simulink library "z5234550RundongGuanLib_DT1_2020"  (R2020a)
settings: Solver=VariableStepAuto  StartTime=0.0  StopTime=10.0  RelTol=1e-3
values from neighbouring files (symbols this model uses):
  Tcs = 1e-4    (= 0.0001)    [z5234550RundongGuanInit_DT1_2020.m]    (also in z5234550RundongGuanSOGIBODE_DT1_2020.m; z5234550RundongGuanTestKiKp_DT1_2020.m; z5234550RundongGuanTestKi_DT1_2020.m; z5234550RundongGuanTestKp_DT1_2020.m)
undefined symbols (not defined in the file or in its folder): DiscIntNeverNeededParam
libraries: $bdroot x6, simulink x5
settings Model: Creator=Kevin  LastModifiedBy=Kevin

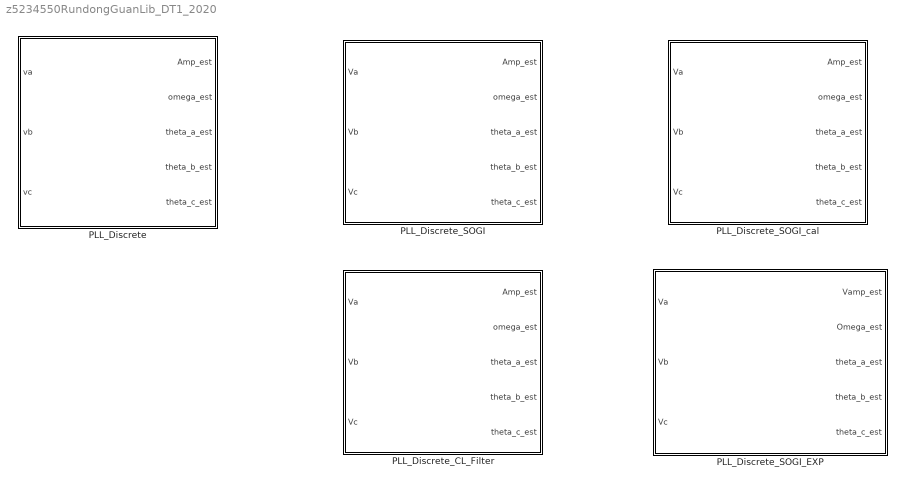
== system z5234550RundongGuanLib_DT1_2020 ==
  PLL_Discrete : Subsystem
  PLL_Discrete_CL_Filter : Subsystem
  PLL_Discrete_SOGI : Subsystem
  PLL_Discrete_SOGI_EXP : Subsystem
  PLL_Discrete_SOGI_cal : Subsystem

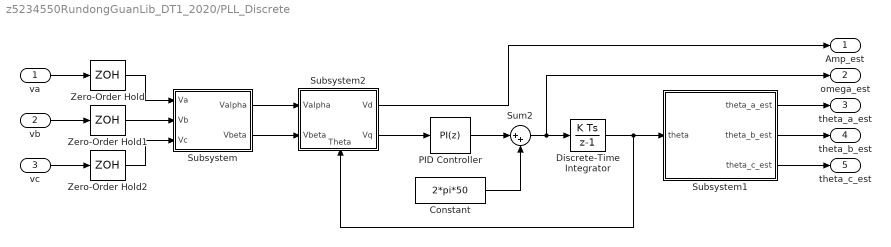
== system z5234550RundongGuanLib_DT1_2020/PLL_Discrete ==
  va : Inport
  vb : Inport  Port=2
  vc : Inport  Port=3
  Constant : Constant  Value=2*pi*50  SampleTime=Tcs
  Discrete-Time Integrator : DiscreteIntegrator  SampleTime=Tcs  ICPrevOutput=DiscIntNeverNeededParam  ICPrevScaledInput=DiscIntNeverNeededParam
  PID Controller : simulink/Continuous/PID Controller  Controller=PI  Form=Parallel  TimeDomain=Discrete-time  UseExternalTs=off  SampleTime=Tcs  IntegratorMethod=Forward Euler  FilterMethod=Forward Euler  ControllerParametersSource=internal  P=4.1744  I=2322.32  D=0  UseFilter=on  N=100  TunerSelectOption=Transfer Function Based (PID Tuner App)  InitialConditionSource=internal  InitialConditionForIntegrator=0  InitialConditionForFilter=0  DifferentiatorICPrevScaledInput=0  ExternalReset=none  TrackingMode=off  Kt=1  LimitOutput=off  UpperSaturationLimit=inf  LowerSaturationLimit=-inf  LinearizeAsGain=on  AntiWindupMode=none  Kb=1  POutMin=[]  POutMax=[]  IOutMin=[]  IOutMax=[]  DOutMin=[]  DOutMax=[]  NOutMin=[]  NOutMax=[]  SumOutMin=[]  SumOutMax=[]  SaturationOutMin=[]  SaturationOutMax=[]  PParamMin=[]  PParamMax=[]  IParamMin=[]  IParamMax=[]  DParamMin=[]  DParamMax=[]  NParamMin=[]  NParamMax=[]  KbParamMin=[]  KbParamMax=[]  KtParamMin=[]  KtParamMax=[]  KbOutMin=[]  KbOutMax=[]  KtOutMin=[]  KtOutMax=[]  IntegratorOutMin=[]  IntegratorOutMax=[]  FilterOutMin=[]  FilterOutMax=[]  SumI1OutMin=[]  SumI1OutMax=[]  SumI2OutMin=[]  SumI2OutMax=[]  SumI3OutMin=[]  SumI3OutMax=[]  SumI4OutMin=[]  SumI4OutMax=[]  SumDOutMin=[]  SumDOutMax=[]  DifferentiatorOutMin=[]  DifferentiatorOutMax=[]  FilterDiffOutCoefMin=[]  FilterDiffOutCoefMax=[]  ReciprocalOutMin=[]  ReciprocalOutMax=[]  SumDenOutMin=[]  SumDenOutMax=[]  SumNumOutMin=[]  SumNumOutMax=[]  DivideOutMin=[]  DivideOutMax=[]  UdiffTsProdOutMin=[]  UdiffTsProdOutMax=[]  NTsProdOutMin=[]  NTsProdOutMax=[]  UintegralTsProdOutMin=[]  UintegralTsProdOutMax=[]  UngainTsProdOutMin=[]  UngainTsProdOutMax=[]  IntegratorContinuousStateAttributes=''  IntegratorStateMustResolveToSignalObject=off  IntegratorRTWStateStorageClass=Auto  FilterContinuousStateAttributes=''  FilterStateMustResolveToSignalObject=off  FilterRTWStateStorageClass=Auto  ParallelPVariant=InternalParameters  IdealPVariant=Disabled  IVariant=InternalParameters  DVariant=Disabled  IntegratorVariant=Discrete  SatVariant=Disabled  AWVariant=Passthrough  PCopyVariant=Disabled  TRVariant=Disabled  FdbkBlocksVariant=Forward  IdealPFdbkVariant=Disabled  SatFdbkVariant=Disabled  DerivativeFilterVariant=Disabled  NVariant=Disabled  NCopyVariant=Disabled_SignalSpec  FilterICVariant=Disabled  IntegratorICVariant=InternalICs  ExternalResetVariant=Disabled  TRSumVariant=Passthrough  SumFdbkVariant=Disabled  SumVariant=Sum_PI  TsampFilterVariant=InternalTs  TsampNgainVariant=Passthrough  TsampIntegralVariant=Passthrough
  Subsystem : Subsystem
  Subsystem1 : Subsystem
  Subsystem2 : Subsystem
      settings: PortSchema="{\"entries\":[{\"content\":{\"sides\":[{\"content\":{\"connectorIds\":[\"In1\",\"In2\"]},\"type\":\"ConnectorPlacement.EquallySpacedRectSide\",\"uuid\":\"d7ee73cc-3741-4077-b32c-689f2c701f83\"},{\"content\":{\"connectorIds\":[\"Out1\",\"Out2\"],\"side\":\"RIGHT\"},\"type\":\"ConnectorPlacement.EquallySpacedRectSide\",\"uuid\":\"fa84044a-ecd8-49d8-a4b2-ae549d89fe8f\"},{\"content\":{\"connectorIds\":[],\"side\":\"TOP\"},\"type\":\"ConnectorPlacement.EquallySpacedRectSide\",\"uuid\":\"692e7773-1833-4597-a5fd-7846ecf4550e\"},{\"content\":{\"connectorIds\":[\"In3\"],\"side\":\"BOTTOM\"},\"type\":\"ConnectorPlacement.EquallySpacedRectSide\",\"uuid\":\"73d654b9-9f56-4244-9824-eb13bf44a38f\"}]},\"type\":\"ConnectorPlacement.EquallySpacedConnector\",\"uuid\":\"4e0b4972-389e-416e-b0d9-9fdc8ba0f1f7\"}],\"packageUris\":[\"http://schema.mathworks.com/mf0/Connector/19700101\"],\"version\":\"1.0\"}"
  Sum2 : Sum  Inputs=|++
  Zero-Order Hold : ZeroOrderHold  SampleTime=Tcs
  Zero-Order Hold1 : ZeroOrderHold  SampleTime=Tcs
  Zero-Order Hold2 : ZeroOrderHold  SampleTime=Tcs
  Amp_est : Outport
  omega_est : Outport  Port=2
  theta_a_est : Outport  Port=3
  theta_b_est : Outport  Port=4
  theta_c_est : Outport  Port=5
  wires:
  va/1 -> Zero-Order Hold/1
  vb/1 -> Zero-Order Hold1/1
  vc/1 -> Zero-Order Hold2/1
  Zero-Order Hold/1 -> Subsystem/1(Va)
  Zero-Order Hold2/1 -> Subsystem/3(Vc)
  Zero-Order Hold1/1 -> Subsystem/2(Vb)
  Subsystem/2(Vbeta) -> Subsystem2/2(Vbeta)
  Subsystem/1(Valpha) -> Subsystem2/1(Valpha)
  PID Controller/1 -> Sum2/1
  Subsystem2/1(Vd) -> Amp_est/1
  Constant/1 -> Sum2/2
  Subsystem1/1(theta_a_est) -> theta_a_est/1
  Subsystem1/2(theta_b_est) -> theta_b_est/1
  Subsystem1/3(theta_c_est) -> theta_c_est/1
  Subsystem2/2(Vq) -> PID Controller/1
  Sum2/1 -> Discrete-Time Integrator/1, omega_est/1
  Discrete-Time Integrator/1 -> Subsystem1/1(theta), Subsystem2/3(Theta)

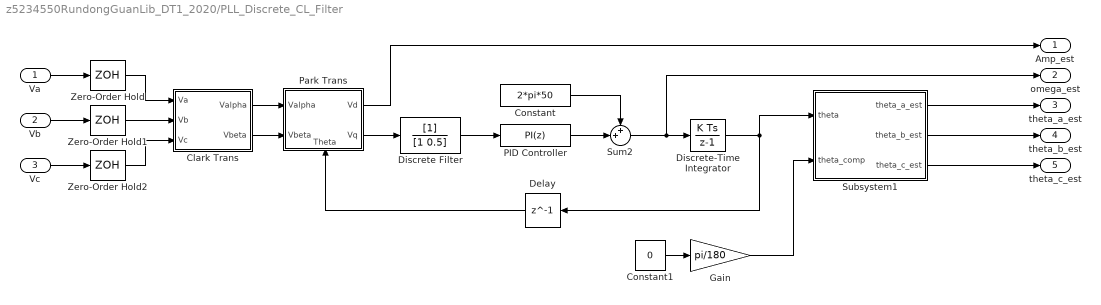
== system z5234550RundongGuanLib_DT1_2020/PLL_Discrete_CL_Filter ==
  Va : Inport
  Vb : Inport  Port=2
  Vc : Inport  Port=3
  Clark Trans : Subsystem
  Constant : Constant  Value=2*pi*50  SampleTime=Tcs
  Constant1 : Constant  Value=0
  Delay : Delay  DelayLength=1  SampleTime=Tcs
  Discrete Filter : DiscreteFilter
  Discrete-Time Integrator : DiscreteIntegrator  SampleTime=Tcs  ICPrevOutput=DiscIntNeverNeededParam  ICPrevScaledInput=DiscIntNeverNeededParam
  Gain : Gain  Gain=pi/180
  PID Controller : simulink/Continuous/PID Controller  Controller=PI  Form=Parallel  TimeDomain=Discrete-time  UseExternalTs=off  SampleTime=Tcs  IntegratorMethod=Forward Euler  FilterMethod=Forward Euler  ControllerParametersSource=internal  P=5.1744  I=0.01  D=0  UseFilter=on  N=100  TunerSelectOption=Transfer Function Based (PID Tuner App)  InitialConditionSource=internal  InitialConditionForIntegrator=0  InitialConditionForFilter=0  DifferentiatorICPrevScaledInput=0  ExternalReset=none  TrackingMode=off  Kt=1  LimitOutput=off  UpperSaturationLimit=inf  LowerSaturationLimit=-inf  LinearizeAsGain=on  AntiWindupMode=none  Kb=1  POutMin=[]  POutMax=[]  IOutMin=[]  IOutMax=[]  DOutMin=[]  DOutMax=[]  NOutMin=[]  NOutMax=[]  SumOutMin=[]  SumOutMax=[]  SaturationOutMin=[]  SaturationOutMax=[]  PParamMin=[]  PParamMax=[]  IParamMin=[]  IParamMax=[]  DParamMin=[]  DParamMax=[]  NParamMin=[]  NParamMax=[]  KbParamMin=[]  KbParamMax=[]  KtParamMin=[]  KtParamMax=[]  KbOutMin=[]  KbOutMax=[]  KtOutMin=[]  KtOutMax=[]  IntegratorOutMin=[]  IntegratorOutMax=[]  FilterOutMin=[]  FilterOutMax=[]  SumI1OutMin=[]  SumI1OutMax=[]  SumI2OutMin=[]  SumI2OutMax=[]  SumI3OutMin=[]  SumI3OutMax=[]  SumI4OutMin=[]  SumI4OutMax=[]  SumDOutMin=[]  SumDOutMax=[]  DifferentiatorOutMin=[]  DifferentiatorOutMax=[]  FilterDiffOutCoefMin=[]  FilterDiffOutCoefMax=[]  ReciprocalOutMin=[]  ReciprocalOutMax=[]  SumDenOutMin=[]  SumDenOutMax=[]  SumNumOutMin=[]  SumNumOutMax=[]  DivideOutMin=[]  DivideOutMax=[]  UdiffTsProdOutMin=[]  UdiffTsProdOutMax=[]  NTsProdOutMin=[]  NTsProdOutMax=[]  UintegralTsProdOutMin=[]  UintegralTsProdOutMax=[]  UngainTsProdOutMin=[]  UngainTsProdOutMax=[]  IntegratorContinuousStateAttributes=''  IntegratorStateMustResolveToSignalObject=off  IntegratorRTWStateStorageClass=Auto  FilterContinuousStateAttributes=''  FilterStateMustResolveToSignalObject=off  FilterRTWStateStorageClass=Auto  ParallelPVariant=InternalParameters  IdealPVariant=Disabled  IVariant=InternalParameters  DVariant=Disabled  IntegratorVariant=Discrete  SatVariant=Disabled  AWVariant=Passthrough  PCopyVariant=Disabled  TRVariant=Disabled  FdbkBlocksVariant=Forward  IdealPFdbkVariant=Disabled  SatFdbkVariant=Disabled  DerivativeFilterVariant=Disabled  NVariant=Disabled  NCopyVariant=Disabled_SignalSpec  FilterICVariant=Disabled  IntegratorICVariant=InternalICs  ExternalResetVariant=Disabled  TRSumVariant=Passthrough  SumFdbkVariant=Disabled  SumVariant=Sum_PI  TsampFilterVariant=InternalTs  TsampNgainVariant=Passthrough  TsampIntegralVariant=Passthrough
  Park Trans : Subsystem
      settings: PortSchema="{\"entries\":[{\"content\":{\"sides\":[{\"content\":{\"connectorIds\":[\"In1\",\"In2\"]},\"type\":\"ConnectorPlacement.EquallySpacedRectSide\",\"uuid\":\"d7ee73cc-3741-4077-b32c-689f2c701f83\"},{\"content\":{\"connectorIds\":[\"Out1\",\"Out2\"],\"side\":\"RIGHT\"},\"type\":\"ConnectorPlacement.EquallySpacedRectSide\",\"uuid\":\"fa84044a-ecd8-49d8-a4b2-ae549d89fe8f\"},{\"content\":{\"connectorIds\":[],\"side\":\"TOP\"},\"type\":\"ConnectorPlacement.EquallySpacedRectSide\",\"uuid\":\"692e7773-1833-4597-a5fd-7846ecf4550e\"},{\"content\":{\"connectorIds\":[\"In3\"],\"side\":\"BOTTOM\"},\"type\":\"ConnectorPlacement.EquallySpacedRectSide\",\"uuid\":\"73d654b9-9f56-4244-9824-eb13bf44a38f\"}]},\"type\":\"ConnectorPlacement.EquallySpacedConnector\",\"uuid\":\"4e0b4972-389e-416e-b0d9-9fdc8ba0f1f7\"}],\"packageUris\":[\"http://schema.mathworks.com/mf0/Connector/19700101\"],\"version\":\"1.0\"}"
  Subsystem1 : Subsystem
  Sum2 : Sum  Inputs=++|
  Zero-Order Hold : ZeroOrderHold  SampleTime=Tcs
  Zero-Order Hold1 : ZeroOrderHold  SampleTime=Tcs
  Zero-Order Hold2 : ZeroOrderHold  SampleTime=Tcs
  Amp_est : Outport
  omega_est : Outport  Port=2
  theta_a_est : Outport  Port=3
  theta_b_est : Outport  Port=4
  theta_c_est : Outport  Port=5
  wires:
  Zero-Order Hold1/1 -> Clark Trans/2(Vb)
  Vc/1 -> Zero-Order Hold2/1
  Vb/1 -> Zero-Order Hold1/1
  Zero-Order Hold2/1 -> Clark Trans/3(Vc)
  Zero-Order Hold/1 -> Clark Trans/1(Va)
  Va/1 -> Zero-Order Hold/1
  Subsystem1/1(theta_a_est) -> theta_a_est/1
  Subsystem1/2(theta_b_est) -> theta_b_est/1
  Subsystem1/3(theta_c_est) -> theta_c_est/1
  Sum2/1 -> Discrete-Time Integrator/1, omega_est/1
  Clark Trans/1(Valpha) -> Park Trans/1(Valpha)
  Clark Trans/2(Vbeta) -> Park Trans/2(Vbeta)
  Delay/1 -> Park Trans/3(Theta)
  PID Controller/1 -> Sum2/2
  Constant/1 -> Sum2/1
  Discrete-Time Integrator/1 -> Subsystem1/1(theta), Delay/1
  Park Trans/1(Vd) -> Amp_est/1
  Constant1/1 -> Gain/1
  Gain/1 -> Subsystem1/2(theta_comp)
  Park Trans/2(Vq) -> Discrete Filter/1
  Discrete Filter/1 -> PID Controller/1

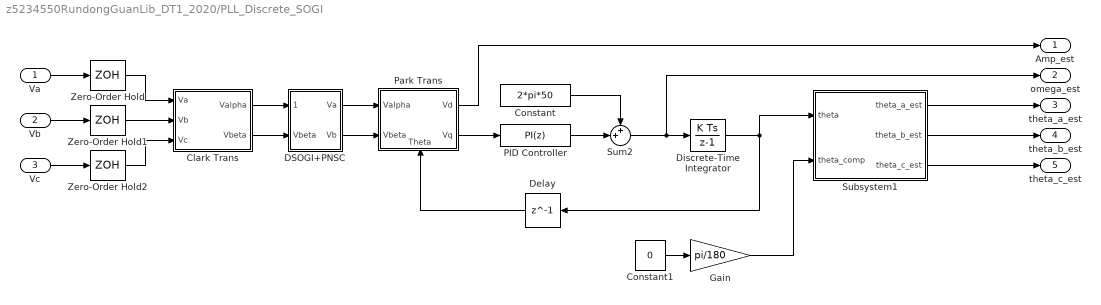
== system z5234550RundongGuanLib_DT1_2020/PLL_Discrete_SOGI ==
  Va : Inport
  Vb : Inport  Port=2
  Vc : Inport  Port=3
  Clark Trans : Subsystem
  Constant : Constant  Value=2*pi*50  SampleTime=Tcs
  Constant1 : Constant  Value=0
  DSOGI+PNSC : Subsystem
  Delay : Delay  DelayLength=1  SampleTime=Tcs
  Discrete-Time Integrator : DiscreteIntegrator  SampleTime=Tcs  ICPrevOutput=DiscIntNeverNeededParam  ICPrevScaledInput=DiscIntNeverNeededParam
  Gain : Gain  Gain=pi/180
  PID Controller : simulink/Continuous/PID Controller  Controller=PI  Form=Parallel  TimeDomain=Discrete-time  UseExternalTs=off  SampleTime=Tcs  IntegratorMethod=Forward Euler  FilterMethod=Forward Euler  ControllerParametersSource=internal  P=5.1744  I=100  D=0  UseFilter=on  N=100  TunerSelectOption=Transfer Function Based (PID Tuner App)  InitialConditionSource=internal  InitialConditionForIntegrator=0  InitialConditionForFilter=0  DifferentiatorICPrevScaledInput=0  ExternalReset=none  TrackingMode=off  Kt=1  LimitOutput=off  UpperSaturationLimit=inf  LowerSaturationLimit=-inf  LinearizeAsGain=on  AntiWindupMode=none  Kb=1  POutMin=[]  POutMax=[]  IOutMin=[]  IOutMax=[]  DOutMin=[]  DOutMax=[]  NOutMin=[]  NOutMax=[]  SumOutMin=[]  SumOutMax=[]  SaturationOutMin=[]  SaturationOutMax=[]  PParamMin=[]  PParamMax=[]  IParamMin=[]  IParamMax=[]  DParamMin=[]  DParamMax=[]  NParamMin=[]  NParamMax=[]  KbParamMin=[]  KbParamMax=[]  KtParamMin=[]  KtParamMax=[]  KbOutMin=[]  KbOutMax=[]  KtOutMin=[]  KtOutMax=[]  IntegratorOutMin=[]  IntegratorOutMax=[]  FilterOutMin=[]  FilterOutMax=[]  SumI1OutMin=[]  SumI1OutMax=[]  SumI2OutMin=[]  SumI2OutMax=[]  SumI3OutMin=[]  SumI3OutMax=[]  SumI4OutMin=[]  SumI4OutMax=[]  SumDOutMin=[]  SumDOutMax=[]  DifferentiatorOutMin=[]  DifferentiatorOutMax=[]  FilterDiffOutCoefMin=[]  FilterDiffOutCoefMax=[]  ReciprocalOutMin=[]  ReciprocalOutMax=[]  SumDenOutMin=[]  SumDenOutMax=[]  SumNumOutMin=[]  SumNumOutMax=[]  DivideOutMin=[]  DivideOutMax=[]  UdiffTsProdOutMin=[]  UdiffTsProdOutMax=[]  NTsProdOutMin=[]  NTsProdOutMax=[]  UintegralTsProdOutMin=[]  UintegralTsProdOutMax=[]  UngainTsProdOutMin=[]  UngainTsProdOutMax=[]  IntegratorContinuousStateAttributes=''  IntegratorStateMustResolveToSignalObject=off  IntegratorRTWStateStorageClass=Auto  FilterContinuousStateAttributes=''  FilterStateMustResolveToSignalObject=off  FilterRTWStateStorageClass=Auto  ParallelPVariant=InternalParameters  IdealPVariant=Disabled  IVariant=InternalParameters  DVariant=Disabled  IntegratorVariant=Discrete  SatVariant=Disabled  AWVariant=Passthrough  PCopyVariant=Disabled  TRVariant=Disabled  FdbkBlocksVariant=Forward  IdealPFdbkVariant=Disabled  SatFdbkVariant=Disabled  DerivativeFilterVariant=Disabled  NVariant=Disabled  NCopyVariant=Disabled_SignalSpec  FilterICVariant=Disabled  IntegratorICVariant=InternalICs  ExternalResetVariant=Disabled  TRSumVariant=Passthrough  SumFdbkVariant=Disabled  SumVariant=Sum_PI  TsampFilterVariant=InternalTs  TsampNgainVariant=Passthrough  TsampIntegralVariant=Passthrough
  Park Trans : Subsystem
      settings: PortSchema="{\"entries\":[{\"content\":{\"sides\":[{\"content\":{\"connectorIds\":[\"In1\",\"In2\"]},\"type\":\"ConnectorPlacement.EquallySpacedRectSide\",\"uuid\":\"d7ee73cc-3741-4077-b32c-689f2c701f83\"},{\"content\":{\"connectorIds\":[\"Out1\",\"Out2\"],\"side\":\"RIGHT\"},\"type\":\"ConnectorPlacement.EquallySpacedRectSide\",\"uuid\":\"fa84044a-ecd8-49d8-a4b2-ae549d89fe8f\"},{\"content\":{\"connectorIds\":[],\"side\":\"TOP\"},\"type\":\"ConnectorPlacement.EquallySpacedRectSide\",\"uuid\":\"692e7773-1833-4597-a5fd-7846ecf4550e\"},{\"content\":{\"connectorIds\":[\"In3\"],\"side\":\"BOTTOM\"},\"type\":\"ConnectorPlacement.EquallySpacedRectSide\",\"uuid\":\"73d654b9-9f56-4244-9824-eb13bf44a38f\"}]},\"type\":\"ConnectorPlacement.EquallySpacedConnector\",\"uuid\":\"4e0b4972-389e-416e-b0d9-9fdc8ba0f1f7\"}],\"packageUris\":[\"http://schema.mathworks.com/mf0/Connector/19700101\"],\"version\":\"1.0\"}"
  Subsystem1 : Subsystem
  Sum2 : Sum  Inputs=++|
  Zero-Order Hold : ZeroOrderHold  SampleTime=Tcs
  Zero-Order Hold1 : ZeroOrderHold  SampleTime=Tcs
  Zero-Order Hold2 : ZeroOrderHold  SampleTime=Tcs
  Amp_est : Outport
  omega_est : Outport  Port=2
  theta_a_est : Outport  Port=3
  theta_b_est : Outport  Port=4
  theta_c_est : Outport  Port=5
  wires:
  Zero-Order Hold1/1 -> Clark Trans/2(Vb)
  Vc/1 -> Zero-Order Hold2/1
  Vb/1 -> Zero-Order Hold1/1
  Zero-Order Hold2/1 -> Clark Trans/3(Vc)
  Zero-Order Hold/1 -> Clark Trans/1(Va)
  Va/1 -> Zero-Order Hold/1
  Subsystem1/1(theta_a_est) -> theta_a_est/1
  Subsystem1/2(theta_b_est) -> theta_b_est/1
  Subsystem1/3(theta_c_est) -> theta_c_est/1
  Sum2/1 -> Discrete-Time Integrator/1, omega_est/1
  Park Trans/2(Vq) -> PID Controller/1
  Clark Trans/1(Valpha) -> DSOGI+PNSC/1(Valpha)
  Clark Trans/2(Vbeta) -> DSOGI+PNSC/2(Vbeta)
  DSOGI+PNSC/1(Va) -> Park Trans/1(Valpha)
  DSOGI+PNSC/2(Vb) -> Park Trans/2(Vbeta)
  Delay/1 -> Park Trans/3(Theta)
  PID Controller/1 -> Sum2/2
  Constant/1 -> Sum2/1
  Discrete-Time Integrator/1 -> Subsystem1/1(theta), Delay/1
  Park Trans/1(Vd) -> Amp_est/1
  Constant1/1 -> Gain/1
  Gain/1 -> Subsystem1/2(theta_comp)

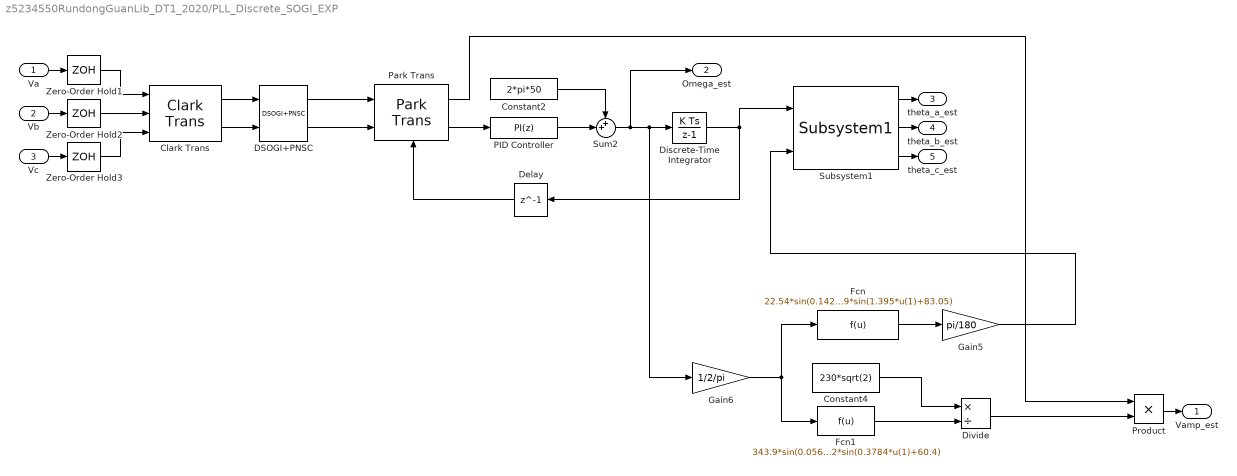
== system z5234550RundongGuanLib_DT1_2020/PLL_Discrete_SOGI_EXP ==
  Va : Inport
  Vb : Inport  Port=2
  Vc : Inport  Port=3
  Clark Trans : $bdroot/PLL_Discrete_SOGI/Clark Trans  SystemSampleTime=-1  Latency=0  AutoFrameSizeCalculation=off
  Constant2 : Constant  Value=2*pi*50  SampleTime=Tcs
  Constant4 : Constant  Value=230*sqrt(2)
  DSOGI+PNSC : $bdroot/PLL_Discrete_SOGI/DSOGI+PNSC  SystemSampleTime=-1  Latency=0  AutoFrameSizeCalculation=off
      link override Subsystem1/Gain: Gain=0.75
      link override Subsystem3/Gain: Gain=0.75
  Delay : Delay  DelayLength=1  SampleTime=Tcs
  Discrete-Time Integrator : DiscreteIntegrator  SampleTime=Tcs  ICPrevOutput=DiscIntNeverNeededParam  ICPrevScaledInput=DiscIntNeverNeededParam
  Divide : Product  Inputs=*/
  Fcn : Fcn  Expr=22.54*sin(0.1425*u(1)+68.25)+0.07009*sin(1.395*u(1)+83.05)
  Fcn1 : Fcn  Expr=343.9*sin(0.05621*u(1)+36.6)+1.732*sin(0.3784*u(1)+60.4)
  Gain5 : Gain  Gain=pi/180
  Gain6 : Gain  Gain=1/2/pi
  PID Controller : simulink/Continuous/PID Controller  Controller=PI  Form=Parallel  TimeDomain=Discrete-time  UseExternalTs=off  SampleTime=Tcs  IntegratorMethod=Forward Euler  FilterMethod=Forward Euler  ControllerParametersSource=internal  P=4  I=100  D=0  UseFilter=on  N=100  TunerSelectOption=Transfer Function Based (PID Tuner App)  InitialConditionSource=internal  InitialConditionForIntegrator=0  InitialConditionForFilter=0  DifferentiatorICPrevScaledInput=0  ExternalReset=none  TrackingMode=off  Kt=1  LimitOutput=off  UpperSaturationLimit=inf  LowerSaturationLimit=-inf  LinearizeAsGain=on  AntiWindupMode=none  Kb=1  POutMin=[]  POutMax=[]  IOutMin=[]  IOutMax=[]  DOutMin=[]  DOutMax=[]  NOutMin=[]  NOutMax=[]  SumOutMin=[]  SumOutMax=[]  SaturationOutMin=[]  SaturationOutMax=[]  PParamMin=[]  PParamMax=[]  IParamMin=[]  IParamMax=[]  DParamMin=[]  DParamMax=[]  NParamMin=[]  NParamMax=[]  KbParamMin=[]  KbParamMax=[]  KtParamMin=[]  KtParamMax=[]  KbOutMin=[]  KbOutMax=[]  KtOutMin=[]  KtOutMax=[]  IntegratorOutMin=[]  IntegratorOutMax=[]  FilterOutMin=[]  FilterOutMax=[]  SumI1OutMin=[]  SumI1OutMax=[]  SumI2OutMin=[]  SumI2OutMax=[]  SumI3OutMin=[]  SumI3OutMax=[]  SumI4OutMin=[]  SumI4OutMax=[]  SumDOutMin=[]  SumDOutMax=[]  DifferentiatorOutMin=[]  DifferentiatorOutMax=[]  FilterDiffOutCoefMin=[]  FilterDiffOutCoefMax=[]  ReciprocalOutMin=[]  ReciprocalOutMax=[]  SumDenOutMin=[]  SumDenOutMax=[]  SumNumOutMin=[]  SumNumOutMax=[]  DivideOutMin=[]  DivideOutMax=[]  UdiffTsProdOutMin=[]  UdiffTsProdOutMax=[]  NTsProdOutMin=[]  NTsProdOutMax=[]  UintegralTsProdOutMin=[]  UintegralTsProdOutMax=[]  UngainTsProdOutMin=[]  UngainTsProdOutMax=[]  IntegratorContinuousStateAttributes=''  IntegratorStateMustResolveToSignalObject=off  IntegratorRTWStateStorageClass=Auto  FilterContinuousStateAttributes=''  FilterStateMustResolveToSignalObject=off  FilterRTWStateStorageClass=Auto  ParallelPVariant=InternalParameters  IdealPVariant=Disabled  IVariant=InternalParameters  DVariant=Disabled  IntegratorVariant=Discrete  SatVariant=Disabled  AWVariant=Passthrough  PCopyVariant=Disabled  TRVariant=Disabled  FdbkBlocksVariant=Forward  IdealPFdbkVariant=Disabled  SatFdbkVariant=Disabled  DerivativeFilterVariant=Disabled  NVariant=Disabled  NCopyVariant=Disabled_SignalSpec  FilterICVariant=Disabled  IntegratorICVariant=InternalICs  ExternalResetVariant=Disabled  TRSumVariant=Passthrough  SumFdbkVariant=Disabled  SumVariant=Sum_PI  TsampFilterVariant=InternalTs  TsampNgainVariant=Passthrough  TsampIntegralVariant=Passthrough
  Park Trans : $bdroot/PLL_Discrete_SOGI/Park Trans  SystemSampleTime=-1  Latency=0  AutoFrameSizeCalculation=off
      settings: PortSchema="{\"entries\":[{\"content\":{\"sides\":[{\"content\":{\"connectorIds\":[\"In1\",\"In2\"]},\"type\":\"ConnectorPlacement.EquallySpacedRectSide\",\"uuid\":\"d7ee73cc-3741-4077-b32c-689f2c701f83\"},{\"content\":{\"connectorIds\":[\"Out1\",\"Out2\"],\"side\":\"RIGHT\"},\"type\":\"ConnectorPlacement.EquallySpacedRectSide\",\"uuid\":\"fa84044a-ecd8-49d8-a4b2-ae549d89fe8f\"},{\"content\":{\"connectorIds\":[],\"side\":\"TOP\"},\"type\":\"ConnectorPlacement.EquallySpacedRectSide\",\"uuid\":\"692e7773-1833-4597-a5fd-7846ecf4550e\"},{\"content\":{\"connectorIds\":[\"In3\"],\"side\":\"BOTTOM\"},\"type\":\"ConnectorPlacement.EquallySpacedRectSide\",\"uuid\":\"73d654b9-9f56-4244-9824-eb13bf44a38f\"}]},\"type\":\"ConnectorPlacement.EquallySpacedConnector\",\"uuid\":\"4e0b4972-389e-416e-b0d9-9fdc8ba0f1f7\"}],\"packageUris\":[\"http://schema.mathworks.com/mf0/Connector/19700101\"],\"version\":\"1.0\"}"
  Product : Product
  Subsystem1 : $bdroot/PLL_Discrete_SOGI/Subsystem1  SystemSampleTime=-1  Latency=0  AutoFrameSizeCalculation=off
  Sum2 : Sum  Inputs=++|
  Zero-Order Hold1 : ZeroOrderHold  SampleTime=Tcs
  Zero-Order Hold2 : ZeroOrderHold  SampleTime=Tcs
  Zero-Order Hold3 : ZeroOrderHold  SampleTime=Tcs
  Vamp_est : Outport
  Omega_est : Outport  Port=2
  theta_a_est : Outport  Port=3
  theta_b_est : Outport  Port=4
  theta_c_est : Outport  Port=5
  wires:
  Fcn/1 -> Gain5/1
  Gain5/1 -> Subsystem1/2
  Gain6/1 -> Fcn1/1, Fcn/1
  Constant2/1 -> Sum2/1
  Clark Trans/1 -> DSOGI+PNSC/1
  Constant4/1 -> Divide/1
  Fcn1/1 -> Divide/2
  Discrete-Time Integrator/1 -> Subsystem1/1, Delay/1
  Zero-Order Hold1/1 -> Clark Trans/1
  DSOGI+PNSC/1 -> Park Trans/1
  DSOGI+PNSC/2 -> Park Trans/2
  Va/1 -> Zero-Order Hold1/1
  Park Trans/1 -> Product/1
  Zero-Order Hold3/1 -> Clark Trans/3
  PID Controller/1 -> Sum2/2
  Subsystem1/2 -> theta_b_est/1
  Vb/1 -> Zero-Order Hold2/1
  Subsystem1/1 -> theta_a_est/1
  Zero-Order Hold2/1 -> Clark Trans/2
  Sum2/1 -> Omega_est/1, Gain6/1, Discrete-Time Integrator/1
  Clark Trans/2 -> DSOGI+PNSC/2
  Product/1 -> Vamp_est/1
  Delay/1 -> Park Trans/3
  Park Trans/2 -> PID Controller/1
  Divide/1 -> Product/2
  Vc/1 -> Zero-Order Hold3/1
  Subsystem1/3 -> theta_c_est/1

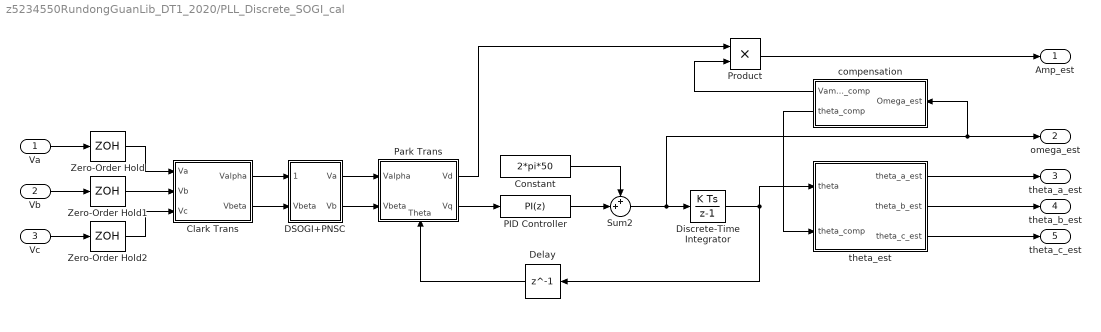
== system z5234550RundongGuanLib_DT1_2020/PLL_Discrete_SOGI_cal ==
  Va : Inport
  Vb : Inport  Port=2
  Vc : Inport  Port=3
  Clark Trans : Subsystem
  Constant : Constant  Value=2*pi*50  SampleTime=Tcs
  DSOGI+PNSC : Subsystem
  Delay : Delay  DelayLength=1  SampleTime=Tcs
  Discrete-Time Integrator : DiscreteIntegrator  SampleTime=Tcs  ICPrevOutput=DiscIntNeverNeededParam  ICPrevScaledInput=DiscIntNeverNeededParam
  PID Controller : simulink/Continuous/PID Controller  Controller=PI  Form=Parallel  TimeDomain=Discrete-time  UseExternalTs=off  SampleTime=Tcs  IntegratorMethod=Forward Euler  FilterMethod=Forward Euler  ControllerParametersSource=internal  P=4  I=100  D=0  UseFilter=on  N=100  TunerSelectOption=Transfer Function Based (PID Tuner App)  InitialConditionSource=internal  InitialConditionForIntegrator=0  InitialConditionForFilter=0  DifferentiatorICPrevScaledInput=0  ExternalReset=none  TrackingMode=off  Kt=1  LimitOutput=off  UpperSaturationLimit=inf  LowerSaturationLimit=-inf  LinearizeAsGain=on  AntiWindupMode=none  Kb=1  POutMin=[]  POutMax=[]  IOutMin=[]  IOutMax=[]  DOutMin=[]  DOutMax=[]  NOutMin=[]  NOutMax=[]  SumOutMin=[]  SumOutMax=[]  SaturationOutMin=[]  SaturationOutMax=[]  PParamMin=[]  PParamMax=[]  IParamMin=[]  IParamMax=[]  DParamMin=[]  DParamMax=[]  NParamMin=[]  NParamMax=[]  KbParamMin=[]  KbParamMax=[]  KtParamMin=[]  KtParamMax=[]  KbOutMin=[]  KbOutMax=[]  KtOutMin=[]  KtOutMax=[]  IntegratorOutMin=[]  IntegratorOutMax=[]  FilterOutMin=[]  FilterOutMax=[]  SumI1OutMin=[]  SumI1OutMax=[]  SumI2OutMin=[]  SumI2OutMax=[]  SumI3OutMin=[]  SumI3OutMax=[]  SumI4OutMin=[]  SumI4OutMax=[]  SumDOutMin=[]  SumDOutMax=[]  DifferentiatorOutMin=[]  DifferentiatorOutMax=[]  FilterDiffOutCoefMin=[]  FilterDiffOutCoefMax=[]  ReciprocalOutMin=[]  ReciprocalOutMax=[]  SumDenOutMin=[]  SumDenOutMax=[]  SumNumOutMin=[]  SumNumOutMax=[]  DivideOutMin=[]  DivideOutMax=[]  UdiffTsProdOutMin=[]  UdiffTsProdOutMax=[]  NTsProdOutMin=[]  NTsProdOutMax=[]  UintegralTsProdOutMin=[]  UintegralTsProdOutMax=[]  UngainTsProdOutMin=[]  UngainTsProdOutMax=[]  IntegratorContinuousStateAttributes=''  IntegratorStateMustResolveToSignalObject=off  IntegratorRTWStateStorageClass=Auto  FilterContinuousStateAttributes=''  FilterStateMustResolveToSignalObject=off  FilterRTWStateStorageClass=Auto  ParallelPVariant=InternalParameters  IdealPVariant=Disabled  IVariant=InternalParameters  DVariant=Disabled  IntegratorVariant=Discrete  SatVariant=Disabled  AWVariant=Passthrough  PCopyVariant=Disabled  TRVariant=Disabled  FdbkBlocksVariant=Forward  IdealPFdbkVariant=Disabled  SatFdbkVariant=Disabled  DerivativeFilterVariant=Disabled  NVariant=Disabled  NCopyVariant=Disabled_SignalSpec  FilterICVariant=Disabled  IntegratorICVariant=InternalICs  ExternalResetVariant=Disabled  TRSumVariant=Passthrough  SumFdbkVariant=Disabled  SumVariant=Sum_PI  TsampFilterVariant=InternalTs  TsampNgainVariant=Passthrough  TsampIntegralVariant=Passthrough
  Park Trans : Subsystem
      settings: PortSchema="{\"entries\":[{\"content\":{\"sides\":[{\"content\":{\"connectorIds\":[\"In1\",\"In2\"]},\"type\":\"ConnectorPlacement.EquallySpacedRectSide\",\"uuid\":\"d7ee73cc-3741-4077-b32c-689f2c701f83\"},{\"content\":{\"connectorIds\":[\"Out1\",\"Out2\"],\"side\":\"RIGHT\"},\"type\":\"ConnectorPlacement.EquallySpacedRectSide\",\"uuid\":\"fa84044a-ecd8-49d8-a4b2-ae549d89fe8f\"},{\"content\":{\"connectorIds\":[],\"side\":\"TOP\"},\"type\":\"ConnectorPlacement.EquallySpacedRectSide\",\"uuid\":\"692e7773-1833-4597-a5fd-7846ecf4550e\"},{\"content\":{\"connectorIds\":[\"In3\"],\"side\":\"BOTTOM\"},\"type\":\"ConnectorPlacement.EquallySpacedRectSide\",\"uuid\":\"73d654b9-9f56-4244-9824-eb13bf44a38f\"}]},\"type\":\"ConnectorPlacement.EquallySpacedConnector\",\"uuid\":\"4e0b4972-389e-416e-b0d9-9fdc8ba0f1f7\"}],\"packageUris\":[\"http://schema.mathworks.com/mf0/Connector/19700101\"],\"version\":\"1.0\"}"
  Product : Product
  Sum2 : Sum  Inputs=++|
  Zero-Order Hold : ZeroOrderHold  SampleTime=Tcs
  Zero-Order Hold1 : ZeroOrderHold  SampleTime=Tcs
  Zero-Order Hold2 : ZeroOrderHold  SampleTime=Tcs
  compensation : Subsystem
      settings: PortSchema="{\"entries\":[{\"content\":{\"sides\":[{\"content\":{\"connectorIds\":[\"Out1\",\"Out2\"]},\"type\":\"ConnectorPlacement.EquallySpacedRectSide\",\"uuid\":\"1da655cf-4ef1-485d-9c9d-29e08b49196c\"},{\"content\":{\"connectorIds\":[\"In1\"],\"side\":\"RIGHT\"},\"type\":\"ConnectorPlacement.EquallySpacedRectSide\",\"uuid\":\"274b50d4-d2b9-4d73-9fa7-29da8dc32335\"},{\"content\":{\"connectorIds\":[],\"side\":\"TOP\"},\"type\":\"ConnectorPlacement.EquallySpacedRectSide\",\"uuid\":\"51928977-61f6-4419-af9c-6bbf4ccbe560\"}]},\"type\":\"ConnectorPlacement.EquallySpacedConnector\",\"uuid\":\"bbbb2fbe-31dd-41e3-8294-b416b392d210\"}],\"packageUris\":[\"http://schema.mathworks.com/mf0/Connector/19700101\"],\"version\":\"1.0\"}"
  theta_est : Subsystem
  Amp_est : Outport
  omega_est : Outport  Port=2
  theta_a_est : Outport  Port=3
  theta_b_est : Outport  Port=4
  theta_c_est : Outport  Port=5
  wires:
  Discrete-Time Integrator/1 -> Delay/1, theta_est/1(theta)
  Constant/1 -> Sum2/1
  PID Controller/1 -> Sum2/2
  Delay/1 -> Park Trans/3(Theta)
  DSOGI+PNSC/2(Vb) -> Park Trans/2(Vbeta)
  DSOGI+PNSC/1(Va) -> Park Trans/1(Valpha)
  Clark Trans/2(Vbeta) -> DSOGI+PNSC/2(Vbeta)
  Clark Trans/1(Valpha) -> DSOGI+PNSC/1(Valpha)
  Park Trans/2(Vq) -> PID Controller/1
  theta_est/3(theta_c_est) -> theta_c_est/1
  theta_est/2(theta_b_est) -> theta_b_est/1
  theta_est/1(theta_a_est) -> theta_a_est/1
  Va/1 -> Zero-Order Hold/1
  Zero-Order Hold/1 -> Clark Trans/1(Va)
  Zero-Order Hold2/1 -> Clark Trans/3(Vc)
  Vb/1 -> Zero-Order Hold1/1
  Vc/1 -> Zero-Order Hold2/1
  Zero-Order Hold1/1 -> Clark Trans/2(Vb)
  Sum2/1 -> compensation/1(Omega_est), omega_est/1, Discrete-Time Integrator/1
  Product/1 -> Amp_est/1
  compensation/1(Vamp_comp) -> Product/2
  Park Trans/1(Vd) -> Product/1
  compensation/2(theta_comp) -> theta_est/2(theta_comp)

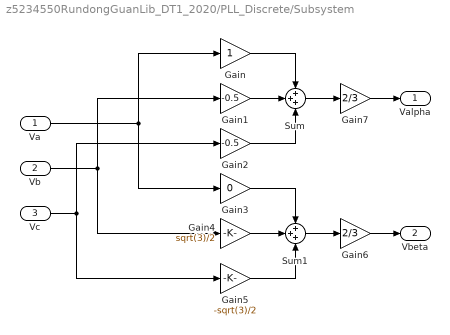
== system z5234550RundongGuanLib_DT1_2020/PLL_Discrete/Subsystem ==
  Va : Inport
  Vb : Inport  Port=2
  Vc : Inport  Port=3
  Gain : Gain
  Gain1 : Gain  Gain=-0.5
  Gain2 : Gain  Gain=-0.5
  Gain3 : Gain  Gain=0
  Gain4 : Gain  Gain=sqrt(3)/2
  Gain5 : Gain  Gain=-sqrt(3)/2
  Gain6 : Gain  Gain=2/3
  Gain7 : Gain  Gain=2/3
  Sum : Sum  Inputs=+++
  Sum1 : Sum  Inputs=+++
  Valpha : Outport
  Vbeta : Outport  Port=2
  wires:
  Gain2/1 -> Sum/3
  Va/1 -> Gain3/1, Gain/1
  Vc/1 -> Gain5/1, Gain2/1
  Vb/1 -> Gain4/1, Gain1/1
  Gain/1 -> Sum/1
  Gain3/1 -> Sum1/1
  Gain1/1 -> Sum/2
  Gain5/1 -> Sum1/3
  Gain4/1 -> Sum1/2
  Sum/1 -> Gain7/1
  Sum1/1 -> Gain6/1
  Gain6/1 -> Vbeta/1
  Gain7/1 -> Valpha/1

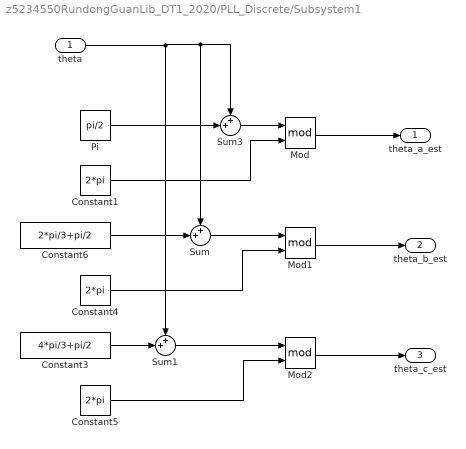
== system z5234550RundongGuanLib_DT1_2020/PLL_Discrete/Subsystem1 ==
  theta : Inport
  Constant1 : Constant  Value=2*pi
  Constant3 : Constant  Value=4*pi/3+pi/2
  Constant4 : Constant  Value=2*pi
  Constant5 : Constant  Value=2*pi
  Constant6 : Constant  Value=2*pi/3+pi/2
  Mod : Math  Operator=mod  SaturateOnIntegerOverflow=on
  Mod1 : Math  Operator=mod  SaturateOnIntegerOverflow=on
  Mod2 : Math  Operator=mod  SaturateOnIntegerOverflow=on
  Pi : Constant  Value=pi/2  OutDataTypeStr=Inherit: Inherit via back propagation
  Sum : Sum  Inputs=++|
  Sum1 : Sum  Inputs=++|
  Sum3 : Sum  Inputs=++|
  theta_a_est : Outport
  theta_b_est : Outport  Port=2
  theta_c_est : Outport  Port=3
  wires:
  Pi/1 -> Sum3/2
  Constant1/1 -> Mod/2
  Constant5/1 -> Mod2/2
  Sum/1 -> Mod1/1
  Sum3/1 -> Mod/1
  Constant3/1 -> Sum1/2
  Constant6/1 -> Sum/2
  Mod/1 -> theta_a_est/1
  theta/1 -> Sum/1, Sum3/1, Sum1/1
  Constant4/1 -> Mod1/2
  Sum1/1 -> Mod2/1
  Mod1/1 -> theta_b_est/1
  Mod2/1 -> theta_c_est/1

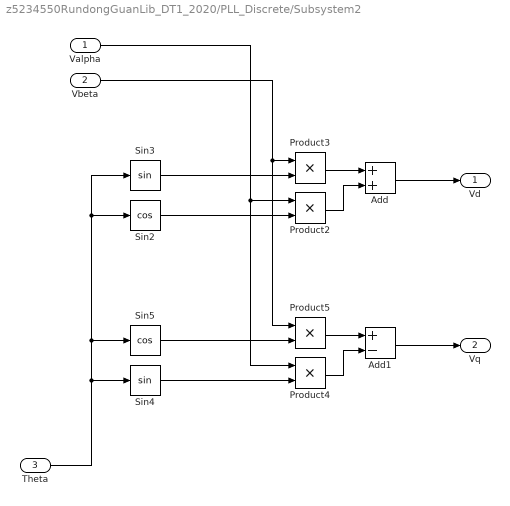
== system z5234550RundongGuanLib_DT1_2020/PLL_Discrete/Subsystem2 ==
  Valpha : Inport
  Vbeta : Inport  Port=2
  Theta : Inport  Port=3
  Add : Sum
  Add1 : Sum  Inputs=+-
  Product{2..5} (4 alike) : Product
  Sin2 : Trigonometry  Operator=cos
  Sin3 : Trigonometry
  Sin4 : Trigonometry
  Sin5 : Trigonometry  Operator=cos
  Vd : Outport
  Vq : Outport  Port=2
  wires:
  Vbeta/1 -> Product5/1, Product3/1
  Theta/1 -> Sin4/1, Sin5/1, Sin2/1, Sin3/1
  Sin5/1 -> Product5/2
  Valpha/1 -> Product2/1, Product4/1
  Product4/1 -> Add1/2
  Product2/1 -> Add/2
  Sin2/1 -> Product2/2
  Add/1 -> Vd/1
  Sin3/1 -> Product3/2
  Product3/1 -> Add/1
  Add1/1 -> Vq/1
  Sin4/1 -> Product4/2
  Product5/1 -> Add1/1

== system z5234550RundongGuanLib_DT1_2020/PLL_Discrete_CL_Filter/Clark Trans ==
  Va : Inport
  Vb : Inport  Port=2
  Vc : Inport  Port=3
  Gain : Gain
  Gain1 : Gain  Gain=-0.5
  Gain2 : Gain  Gain=-0.5
  Gain3 : Gain  Gain=0
  Gain4 : Gain  Gain=sqrt(3)/2
  Gain5 : Gain  Gain=-sqrt(3)/2
  Gain6 : Gain  Gain=2/3
  Gain7 : Gain  Gain=2/3
  Sum : Sum  Inputs=+++
  Sum1 : Sum  Inputs=+++
  Valpha : Outport
  Vbeta : Outport  Port=2
  wires:
  Gain2/1 -> Sum/3
  Va/1 -> Gain3/1, Gain/1
  Vc/1 -> Gain5/1, Gain2/1
  Vb/1 -> Gain4/1, Gain1/1
  Gain/1 -> Sum/1
  Gain3/1 -> Sum1/1
  Gain1/1 -> Sum/2
  Gain5/1 -> Sum1/3
  Gain4/1 -> Sum1/2
  Sum/1 -> Gain7/1
  Sum1/1 -> Gain6/1
  Gain7/1 -> Valpha/1
  Gain6/1 -> Vbeta/1

== system z5234550RundongGuanLib_DT1_2020/PLL_Discrete_CL_Filter/Park Trans ==
  Valpha : Inport
  Vbeta : Inport  Port=2
  Theta : Inport  Port=3
  Add : Sum
  Add1 : Sum  Inputs=+-
  Product{2..5} (4 alike) : Product
  Sin2 : Trigonometry  Operator=cos
  Sin3 : Trigonometry
  Sin4 : Trigonometry
  Sin5 : Trigonometry  Operator=cos
  Vd : Outport
  Vq : Outport  Port=2
  wires:
  Vbeta/1 -> Product5/1, Product3/1
  Theta/1 -> Sin4/1, Sin5/1, Sin2/1, Sin3/1
  Sin5/1 -> Product5/2
  Valpha/1 -> Product2/1, Product4/1
  Product4/1 -> Add1/2
  Product2/1 -> Add/2
  Sin2/1 -> Product2/2
  Add/1 -> Vd/1
  Sin3/1 -> Product3/2
  Product3/1 -> Add/1
  Add1/1 -> Vq/1
  Sin4/1 -> Product4/2
  Product5/1 -> Add1/1

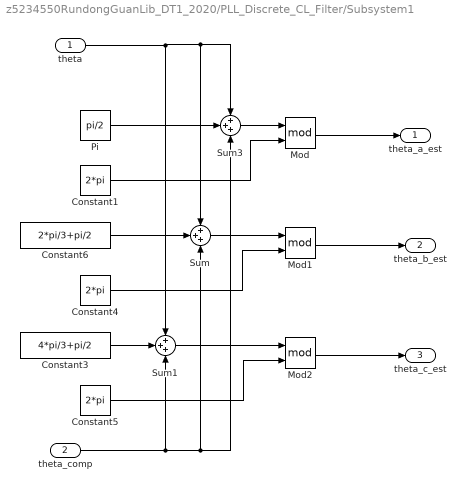
== system z5234550RundongGuanLib_DT1_2020/PLL_Discrete_CL_Filter/Subsystem1 ==
  theta : Inport
  theta_comp : Inport  Port=2
  Constant1 : Constant  Value=2*pi
  Constant3 : Constant  Value=4*pi/3+pi/2
  Constant4 : Constant  Value=2*pi
  Constant5 : Constant  Value=2*pi
  Constant6 : Constant  Value=2*pi/3+pi/2
  Mod : Math  Operator=mod  SaturateOnIntegerOverflow=on
  Mod1 : Math  Operator=mod  SaturateOnIntegerOverflow=on
  Mod2 : Math  Operator=mod  SaturateOnIntegerOverflow=on
  Pi : Constant  Value=pi/2  OutDataTypeStr=Inherit: Inherit via back propagation
  Sum : Sum  Inputs=+++
  Sum1 : Sum  Inputs=+++
  Sum3 : Sum  Inputs=+++
  theta_a_est : Outport
  theta_b_est : Outport  Port=2
  theta_c_est : Outport  Port=3
  wires:
  Mod2/1 -> theta_c_est/1
  Mod1/1 -> theta_b_est/1
  Sum1/1 -> Mod2/1
  Constant4/1 -> Mod1/2
  theta/1 -> Sum1/1, Sum3/1, Sum/1
  Mod/1 -> theta_a_est/1
  Constant6/1 -> Sum/2
  Constant3/1 -> Sum1/2
  Sum3/1 -> Mod/1
  Sum/1 -> Mod1/1
  Constant5/1 -> Mod2/2
  Constant1/1 -> Mod/2
  Pi/1 -> Sum3/2
  theta_comp/1 -> Sum1/3, Sum/3, Sum3/3

== system z5234550RundongGuanLib_DT1_2020/PLL_Discrete_SOGI/Clark Trans ==
  Va : Inport
  Vb : Inport  Port=2
  Vc : Inport  Port=3
  Gain : Gain
  Gain1 : Gain  Gain=-0.5
  Gain2 : Gain  Gain=-0.5
  Gain3 : Gain  Gain=0
  Gain4 : Gain  Gain=sqrt(3)/2
  Gain5 : Gain  Gain=-sqrt(3)/2
  Gain6 : Gain  Gain=2/3
  Gain7 : Gain  Gain=2/3
  Sum : Sum  Inputs=+++
  Sum1 : Sum  Inputs=+++
  Valpha : Outport
  Vbeta : Outport  Port=2
  wires:
  Gain2/1 -> Sum/3
  Va/1 -> Gain3/1, Gain/1
  Vc/1 -> Gain5/1, Gain2/1
  Vb/1 -> Gain4/1, Gain1/1
  Gain/1 -> Sum/1
  Gain3/1 -> Sum1/1
  Gain1/1 -> Sum/2
  Gain5/1 -> Sum1/3
  Gain4/1 -> Sum1/2
  Sum/1 -> Gain7/1
  Sum1/1 -> Gain6/1
  Gain7/1 -> Valpha/1
  Gain6/1 -> Vbeta/1

== system z5234550RundongGuanLib_DT1_2020/PLL_Discrete_SOGI/DSOGI+PNSC ==
  Valpha : Inport
  Vbeta : Inport  Port=2
  Constant : Constant  Value=100*pi
  Gain : Gain  Gain=1/2
  Gain1 : Gain  Gain=1/2
  Gain2 : Gain
  Gain3 : Gain
  Subsystem : Subsystem
  Subsystem1 : $bdroot/PLL_Discrete_SOGI/DSOGI+PNSC/Subsystem3  SystemSampleTime=-1  Latency=0  AutoFrameSizeCalculation=off
  Subsystem3 : Subsystem
  Va : Outport
  Vb : Outport  Port=2
  wires:
  Constant/1 -> Subsystem1/2, Subsystem3/2(Omega0)
  Subsystem3/1(v) -> Subsystem/1(Va')
  Subsystem3/2(qv) -> Subsystem/2(qVa')
  Subsystem/1(Va) -> Gain1/1
  Subsystem/2(Vb) -> Gain/1
  Valpha/1 -> Subsystem3/1(Vg)
  Vbeta/1 -> Subsystem1/1
  Subsystem1/1 -> Subsystem/3(Vb')
  Subsystem1/2 -> Subsystem/4(qVb')
  Gain1/1 -> Gain2/1
  Gain/1 -> Gain3/1
  Gain2/1 -> Va/1
  Gain3/1 -> Vb/1

== system z5234550RundongGuanLib_DT1_2020/PLL_Discrete_SOGI/Park Trans ==
  Valpha : Inport
  Vbeta : Inport  Port=2
  Theta : Inport  Port=3
  Add : Sum
  Add1 : Sum  Inputs=+-
  Product{2..5} (4 alike) : Product
  Sin2 : Trigonometry  Operator=cos
  Sin3 : Trigonometry
  Sin4 : Trigonometry
  Sin5 : Trigonometry  Operator=cos
  Vd : Outport
  Vq : Outport  Port=2
  wires:
  Vbeta/1 -> Product5/1, Product3/1
  Theta/1 -> Sin4/1, Sin5/1, Sin2/1, Sin3/1
  Sin5/1 -> Product5/2
  Valpha/1 -> Product2/1, Product4/1
  Product4/1 -> Add1/2
  Product2/1 -> Add/2
  Sin2/1 -> Product2/2
  Add/1 -> Vd/1
  Sin3/1 -> Product3/2
  Product3/1 -> Add/1
  Add1/1 -> Vq/1
  Sin4/1 -> Product4/2
  Product5/1 -> Add1/1

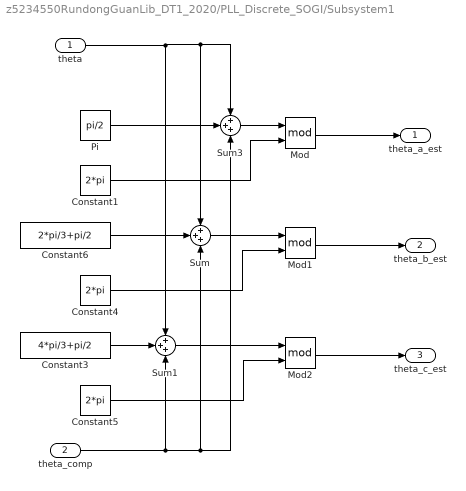
== system z5234550RundongGuanLib_DT1_2020/PLL_Discrete_SOGI/Subsystem1 ==
  theta : Inport
  theta_comp : Inport  Port=2
  Constant1 : Constant  Value=2*pi
  Constant3 : Constant  Value=4*pi/3+pi/2
  Constant4 : Constant  Value=2*pi
  Constant5 : Constant  Value=2*pi
  Constant6 : Constant  Value=2*pi/3+pi/2
  Mod : Math  Operator=mod  SaturateOnIntegerOverflow=on
  Mod1 : Math  Operator=mod  SaturateOnIntegerOverflow=on
  Mod2 : Math  Operator=mod  SaturateOnIntegerOverflow=on
  Pi : Constant  Value=pi/2  OutDataTypeStr=Inherit: Inherit via back propagation
  Sum : Sum  Inputs=+++
  Sum1 : Sum  Inputs=+++
  Sum3 : Sum  Inputs=+++
  theta_a_est : Outport
  theta_b_est : Outport  Port=2
  theta_c_est : Outport  Port=3
  wires:
  Mod2/1 -> theta_c_est/1
  Mod1/1 -> theta_b_est/1
  Sum1/1 -> Mod2/1
  Constant4/1 -> Mod1/2
  theta/1 -> Sum1/1, Sum3/1, Sum/1
  Mod/1 -> theta_a_est/1
  Constant6/1 -> Sum/2
  Constant3/1 -> Sum1/2
  Sum3/1 -> Mod/1
  Sum/1 -> Mod1/1
  Constant5/1 -> Mod2/2
  Constant1/1 -> Mod/2
  Pi/1 -> Sum3/2
  theta_comp/1 -> Sum1/3, Sum/3, Sum3/3

== system z5234550RundongGuanLib_DT1_2020/PLL_Discrete_SOGI_cal/Clark Trans ==
  Va : Inport
  Vb : Inport  Port=2
  Vc : Inport  Port=3
  Gain : Gain
  Gain1 : Gain  Gain=-0.5
  Gain2 : Gain  Gain=-0.5
  Gain3 : Gain  Gain=0
  Gain4 : Gain  Gain=sqrt(3)/2
  Gain5 : Gain  Gain=-sqrt(3)/2
  Gain6 : Gain  Gain=2/3
  Gain7 : Gain  Gain=2/3
  Sum : Sum  Inputs=+++
  Sum1 : Sum  Inputs=+++
  Valpha : Outport
  Vbeta : Outport  Port=2
  wires:
  Gain6/1 -> Vbeta/1
  Gain7/1 -> Valpha/1
  Sum1/1 -> Gain6/1
  Sum/1 -> Gain7/1
  Gain4/1 -> Sum1/2
  Gain5/1 -> Sum1/3
  Gain1/1 -> Sum/2
  Gain3/1 -> Sum1/1
  Gain/1 -> Sum/1
  Vb/1 -> Gain1/1, Gain4/1
  Vc/1 -> Gain2/1, Gain5/1
  Va/1 -> Gain/1, Gain3/1
  Gain2/1 -> Sum/3

== system z5234550RundongGuanLib_DT1_2020/PLL_Discrete_SOGI_cal/DSOGI+PNSC ==
  Valpha : Inport
  Vbeta : Inport  Port=2
  Constant : Constant  Value=100*pi
  Gain : Gain  Gain=1/2
  Gain1 : Gain  Gain=1/2
  Subsystem : Subsystem
  Subsystem1 : $bdroot/PLL_Discrete_SOGI/DSOGI+PNSC/Subsystem3  SystemSampleTime=-1  Latency=0  AutoFrameSizeCalculation=off
      link override Gain: Gain=0.75
  Subsystem3 : Subsystem
  Va : Outport
  Vb : Outport  Port=2
  wires:
  Gain/1 -> Vb/1
  Gain1/1 -> Va/1
  Subsystem1/2 -> Subsystem/4(qVb')
  Subsystem1/1 -> Subsystem/3(Vb')
  Vbeta/1 -> Subsystem1/1
  Valpha/1 -> Subsystem3/1(Vg)
  Subsystem/2(Vb) -> Gain/1
  Subsystem/1(Va) -> Gain1/1
  Subsystem3/2(qv) -> Subsystem/2(qVa')
  Subsystem3/1(v) -> Subsystem/1(Va')
  Constant/1 -> Subsystem3/2(Omega0), Subsystem1/2

== system z5234550RundongGuanLib_DT1_2020/PLL_Discrete_SOGI_cal/Park Trans ==
  Valpha : Inport
  Vbeta : Inport  Port=2
  Theta : Inport  Port=3
  Add : Sum
  Add1 : Sum  Inputs=+-
  Product{2..5} (4 alike) : Product
  Sin2 : Trigonometry  Operator=cos
  Sin3 : Trigonometry
  Sin4 : Trigonometry
  Sin5 : Trigonometry  Operator=cos
  Vd : Outport
  Vq : Outport  Port=2
  wires:
  Product5/1 -> Add1/1
  Sin4/1 -> Product4/2
  Add1/1 -> Vq/1
  Product3/1 -> Add/1
  Sin3/1 -> Product3/2
  Add/1 -> Vd/1
  Sin2/1 -> Product2/2
  Product2/1 -> Add/2
  Product4/1 -> Add1/2
  Valpha/1 -> Product4/1, Product2/1
  Sin5/1 -> Product5/2
  Theta/1 -> Sin3/1, Sin2/1, Sin5/1, Sin4/1
  Vbeta/1 -> Product3/1, Product5/1

== system z5234550RundongGuanLib_DT1_2020/PLL_Discrete_SOGI_cal/compensation ==
  Omega_est : Inport
  Constant4 : Constant  Value=325.08
  Divide : Product  Inputs=*/
  Fcn : Fcn  Expr=22.54*sin(0.1425*u(1)+68.25)+0.07009*sin(1.395*u(1)+83.05)
  Fcn1 : Fcn  Expr=343.9*sin(0.05621*u(1)+36.6)+1.732*sin(0.3784*u(1)+60.4)
  Gain5 : Gain  Gain=pi/180
  Gain6 : Gain  Gain=1/2/pi
  Vamp_comp : Outport
  theta_comp : Outport  Port=2
  wires:
  Fcn1/1 -> Divide/2
  Constant4/1 -> Divide/1
  Fcn/1 -> Gain5/1
  Gain5/1 -> theta_comp/1
  Divide/1 -> Vamp_comp/1
  Omega_est/1 -> Gain6/1
  Gain6/1 -> Fcn1/1, Fcn/1

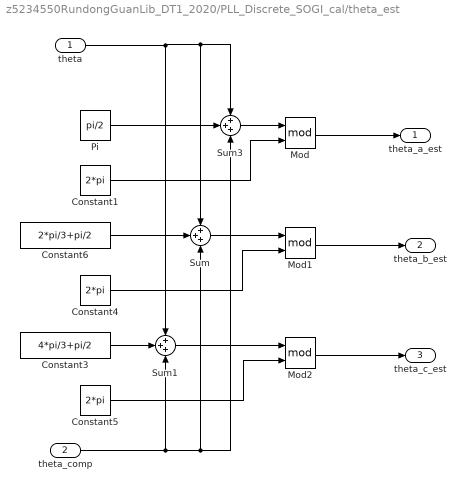
== system z5234550RundongGuanLib_DT1_2020/PLL_Discrete_SOGI_cal/theta_est ==
  theta : Inport
  theta_comp : Inport  Port=2
  Constant1 : Constant  Value=2*pi
  Constant3 : Constant  Value=4*pi/3+pi/2
  Constant4 : Constant  Value=2*pi
  Constant5 : Constant  Value=2*pi
  Constant6 : Constant  Value=2*pi/3+pi/2
  Mod : Math  Operator=mod  SaturateOnIntegerOverflow=on
  Mod1 : Math  Operator=mod  SaturateOnIntegerOverflow=on
  Mod2 : Math  Operator=mod  SaturateOnIntegerOverflow=on
  Pi : Constant  Value=pi/2  OutDataTypeStr=Inherit: Inherit via back propagation
  Sum : Sum  Inputs=+++
  Sum1 : Sum  Inputs=+++
  Sum3 : Sum  Inputs=+++
  theta_a_est : Outport
  theta_b_est : Outport  Port=2
  theta_c_est : Outport  Port=3
  wires:
  theta_comp/1 -> Sum3/3, Sum/3, Sum1/3
  Pi/1 -> Sum3/2
  Constant1/1 -> Mod/2
  Constant5/1 -> Mod2/2
  Sum/1 -> Mod1/1
  Sum3/1 -> Mod/1
  Constant3/1 -> Sum1/2
  Constant6/1 -> Sum/2
  Mod/1 -> theta_a_est/1
  theta/1 -> Sum/1, Sum3/1, Sum1/1
  Constant4/1 -> Mod1/2
  Sum1/1 -> Mod2/1
  Mod1/1 -> theta_b_est/1
  Mod2/1 -> theta_c_est/1

== system z5234550RundongGuanLib_DT1_2020/PLL_Discrete_SOGI/DSOGI+PNSC/Subsystem ==
  Va' : Inport
  qVa' : Inport  Port=2
  Vb' : Inport  Port=3
  qVb' : Inport  Port=4
  Sum : Sum  Inputs=+|-
  Sum1 : Sum  Inputs=+|+
  Va : Outport
  Vb : Outport  Port=2
  wires:
  Sum1/1 -> Vb/1
  Sum/1 -> Va/1
  Va'/1 -> Sum/1
  Vb'/1 -> Sum1/2
  qVa'/1 -> Sum1/1
  qVb'/1 -> Sum/2

== system z5234550RundongGuanLib_DT1_2020/PLL_Discrete_SOGI/DSOGI+PNSC/Subsystem3 ==
  Vg : Inport
  Omega0 : Inport  Port=2
  Discrete-Time Integrator1 : DiscreteIntegrator  SampleTime=Tcs  ICPrevOutput=DiscIntNeverNeededParam  ICPrevScaledInput=DiscIntNeverNeededParam
  Discrete-Time Integrator2 : DiscreteIntegrator  SampleTime=Tcs  ICPrevOutput=DiscIntNeverNeededParam  ICPrevScaledInput=DiscIntNeverNeededParam
  Gain : Gain  Gain=0.8
  Product : Product
  Product1 : Product
  Sum : Sum  Inputs=-+|
  Sum1 : Sum  Inputs=|+-
  v : Outport
  qv : Outport  Port=2
  wires:
  Sum/1 -> Gain/1
  Discrete-Time Integrator1/1 -> v/1, Sum/1, Discrete-Time Integrator2/1
  Omega0/1 -> Product1/2, Product/2
  Product/1 -> Discrete-Time Integrator1/1
  Discrete-Time Integrator2/1 -> Product1/1
  Product1/1 -> qv/1, Sum1/2
  Vg/1 -> Sum/2
  Gain/1 -> Sum1/1
  Sum1/1 -> Product/1

== system z5234550RundongGuanLib_DT1_2020/PLL_Discrete_SOGI_cal/DSOGI+PNSC/Subsystem ==
  Va' : Inport
  qVa' : Inport  Port=2
  Vb' : Inport  Port=3
  qVb' : Inport  Port=4
  Sum : Sum  Inputs=+|-
  Sum1 : Sum  Inputs=+|+
  Va : Outport
  Vb : Outport  Port=2
  wires:
  qVb'/1 -> Sum/2
  qVa'/1 -> Sum1/1
  Vb'/1 -> Sum1/2
  Va'/1 -> Sum/1
  Sum/1 -> Va/1
  Sum1/1 -> Vb/1

== system z5234550RundongGuanLib_DT1_2020/PLL_Discrete_SOGI_cal/DSOGI+PNSC/Subsystem3 ==
  Vg : Inport
  Omega0 : Inport  Port=2
  Discrete-Time Integrator1 : DiscreteIntegrator  SampleTime=Tcs  ICPrevOutput=DiscIntNeverNeededParam  ICPrevScaledInput=DiscIntNeverNeededParam
  Discrete-Time Integrator2 : DiscreteIntegrator  SampleTime=Tcs  ICPrevOutput=DiscIntNeverNeededParam  ICPrevScaledInput=DiscIntNeverNeededParam
  Gain : Gain  Gain=0.75
  Product : Product
  Product1 : Product
  Sum : Sum  Inputs=-+|
  Sum1 : Sum  Inputs=|+-
  v : Outport
  qv : Outport  Port=2
  wires:
  Sum1/1 -> Product/1
  Gain/1 -> Sum1/1
  Vg/1 -> Sum/2
  Product1/1 -> Sum1/2, qv/1
  Discrete-Time Integrator2/1 -> Product1/1
  Product/1 -> Discrete-Time Integrator1/1
  Omega0/1 -> Product/2, Product1/2
  Discrete-Time Integrator1/1 -> Discrete-Time Integrator2/1, Sum/1, v/1
  Sum/1 -> Gain/1
